simulink model "parts"  (R2021b)
settings: Solver=ode15s  StartTime=0.0  StopTime=t_f  MaxStep=max_step_size  RelTol=1e-3
values from neighbouring files (symbols this model uses):
  cont_param_10 = in    [double_pendulum.m]    (also in optimize_10_SMC_single_first_explicit.m = cont_param_10_surrogateopt)
  cont_param_11 = in    [double_pendulum.m]    (also in optimize_11_SMC_single_first_implicit.m = cont_param_11_surrogateopt)
  cont_param_12 = in    [double_pendulum.m]    (also in optimize_12_SMC_single_last_explicit.m = cont_param_12_surrogateopt)
  cont_param_13 = in    [double_pendulum.m]    (also in optimize_13_SMC_single_last_implicit.m = cont_param_13_surrogateopt)
  cont_param_14 = in    [double_pendulum.m]    (also in optimize_14_SMC_double_explicit.m = cont_param_14_surrogateopt)
  cont_param_15 = in    [double_pendulum.m]    (also in optimize_15_SMC_double_implicit.m = cont_param_15_surrogateopt)
  cont_param_16 = in    [double_pendulum.m]
  cont_param_17 = in    [double_pendulum.m]
  cont_param_18 = in    [double_pendulum.m]
  cont_param_19 = in    [double_pendulum.m]
  cont_param_4 = in    [double_pendulum.m]
  cont_param_5 = in    [double_pendulum.m]
  cont_param_6 = in    [double_pendulum.m]
  cont_param_7 = in    [double_pendulum.m]
  cont_param_8 = in    [double_pendulum.m]
  cont_param_9 = in    [double_pendulum.m]
  h = 1e-5    (= 1e-05)    [Conference_paper.m]    (also in Latest.m)
  m = 10    [Conference_paper.m]    (also in Latest.m = 100; control_8_collocated_PD_tracking.m = load_mass+hook_mass+cable_mass_total)
  method_select = Method    [main_run.m]    (also in modify_tracking.m = 3)
  N = floor(t_f / h)    [control_2_zero_vibration.m]    (also in control_3_ZVD.m; modify_tracking.m = 3)
  s = c1*(x-xd)+c2*(v-vd)+c3*theta_dot_1+c4*theta_1    [control_10_SMC_single_first_explicit.m]    (also in control_11_SMC_single_first_implicit.m = c1*(x-xd)+c2*(v-vd)+c3*theta_dot+c4*theta; control_12_SMC_single_last_explicit.m = c1*(x-xd)+c2*(v-vd)+c3*theta_dot_2+c4*theta_2; control_13_SMC_single_last_implicit.m = c1*(x-xd)+c2*(v-vd)+c3*theta_dot+c4*theta; control_14_SMC_double_explicit.m = (v-vd)+lambda*(x-xd)+alpha*theta_1+beta*theta_2)
  X = ex+lambda*sin(theta)    [control_16_PD_energy_first.m]    (also in control_17_PD_energy_last.m)
  Z = cont_param_8(4)    [control_8_collocated_PD_tracking.m]
undefined symbols (not defined in the file or in its folder): a_d_full, all_initial_sway, c_actuator, cable_eact_piece, cable_length, cable_mass_total, cart_disturbance_amp, cart_mass, delay_time, first_link_sway, hook_mass, last_piece_length, load_disturbance_amp, number_of_pendulums, payload_mass, sat_const, t_f, total_mass, traj_number, Y
libraries: sm_lib x72, nesl_utility x47, commchan3 x4
(part 1 of 2)
settings Model: Creator=rmoja  LastModifiedBy=SESA642626

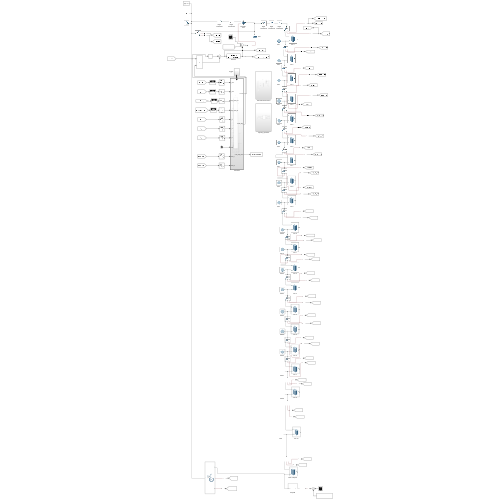
[thumbnail: Simulink's stored preview of the top-level diagram]
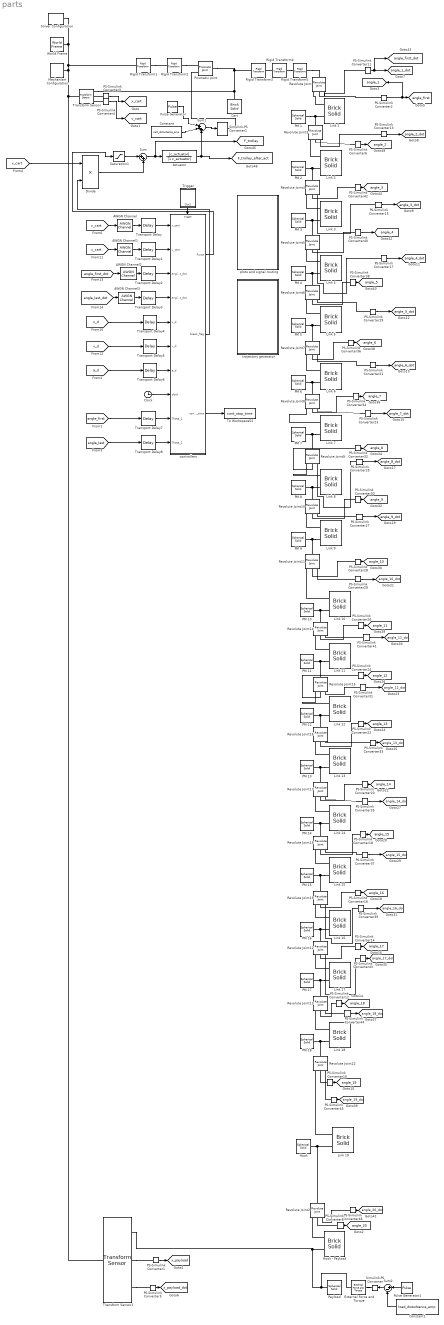
== system parts ==
  AWGN Channel{,1..3} (4 alike) : commchan3/AWGN Channel  InputProcessing=Columns as channels (frame based)  seed=67  noiseMode="Signal to noise ratio  (SNR)"  EbNodB=10  EsNodB=10  SNRdB=SNR_value  bitsPerSym=1  Ps=1  Tsym=1  variance=1
  Actuator : TransferFcn  Numerator=[c_actuator]  Denominator=[1 c_actuator]
  Cart : sm_lib/Body Elements/Brick Solid  GraphicAmbientColor=[0.15 0.15 0.15 1.0]  BasedOnType=Mass  BrickDimensions=[1/2 1/2 1/2]  BrickDimensionUnits=m  CenterOfMass=[0 0 0]  CenterOfMassUnits=m  GraphicDiffuseColor=[0 0 1]  Density=1000  DensityUnits=kg/(m^3)  DoExposeReferenceFrame=on  GraphicEmissiveColor=[0.0 0.0 0.0 1.0]  ExportEntireGeometry=off  SerializedFrames=<Frames/>  MarkerShape=Sphere  MarkerSize=10  GraphicType=FromGeometry  InertiaType=PointMass  Mass=cart_mass  MassUnits=kg  MomentsOfInertia=[1 1 1]  MomentsOfInertiaUnits=kg*m^2  GraphicOpacity=1.0  ProductsOfInertia=[0 0 0]  ProductsOfInertiaUnits=kg*m^2  GraphicShininess=75  GraphicSpecularColor=[0.5 0.5 0.5 1.0]  GraphicVisPropType=SimpleVisualProperties
  Clock : Clock
  Constant : Constant  Value=cart_disturbance_amp
  Constant1 : Constant  Value=load_disturbance_amp
  Divide : Product  Inputs=**
  External Force and Torque : sm_lib/Forces and Torques/External Force and Torque  ForceResolutionFrame=World  EnableForceX=on  EnableForceY=off  EnableForceZ=off  EnableForce=off  TorqueResolutionFrame=AttachedFrame  EnableTorqueX=off  EnableTorqueY=off  EnableTorqueZ=off  EnableTorque=off
  Hook : sm_lib/Body Elements/Spherical Solid  GraphicAmbientColor=[0.15 0.15 0.15 1.0]  BasedOnType=Density  CenterOfMass=[0 0 0]  CenterOfMassUnits=m  GraphicDiffuseColor=[1.0 0.2 0.0]  Density=1000  DensityUnits=kg/(m^3)  DoExposeReferenceFrame=on  GraphicEmissiveColor=[0.0 0.0 0.0 1.0]  ExportEntireGeometry=off  SerializedExposedGeometries=<ExposedGeometries/>  SerializedFrames=<Frames/>  MarkerShape=Sphere  MarkerSize=10  GraphicType=FromGeometry  InertiaType=PointMass  Mass=hook_mass-0.1  MassUnits=kg  MomentsOfInertia=[1 1 1]*1e-3  MomentsOfInertiaUnits=kg*m^2  GraphicOpacity=1.0  ProductsOfInertia=[0 0 0]  ProductsOfInertiaUnits=kg*m^2  GraphicShininess=75  GraphicSpecularColor=[0.5 0.5 0.5 1.0]  SphereRadius=0.2  SphereRadiusUnits=m  GraphicVisPropType=SimpleVisualProperties
  Hook - Payload : sm_lib/Body Elements/Brick Solid  GraphicAmbientColor=[0.15 0.15 0.15 1.0]  BasedOnType=Density  BrickDimensions=[last_piece_length 0.06 0.06]  BrickDimensionUnits=m  CenterOfMass=[0 0 0]  CenterOfMassUnits=m  GraphicDiffuseColor=[0.0 1 0.0]  Density=78000  DensityUnits=kg/m^3  DoExposeReferenceFrame=on  GraphicEmissiveColor=[0.0 0.0 0.0 1.0]  ExportEntireGeometry=off  SerializedFrames=<Frames><Frame><Id>Frame1</Id><Value><Name>F1</Name><Origin><Source>GeometricFeature</Source><FeatureName>-x surface</FeatureName></Origin><PrimaryAxis><DefinedDirection>+Z</DefinedDirection><Source>ReferenceFrame</Source><SourceDirection>+Z</SourceDirection><FeatureName></FeatureName></PrimaryAxis><SecondaryAxis><DefinedDirection>+X</DefinedDirection><Source>ReferenceFrame</Source><SourceDirection>+X</SourceDirection><FeatureName></FeatureName></SecondaryAxis></Value></Frame><Frame><Id>Frame2</Id><Value><Name>F2</Name><Origin><Source>GeometricFeature</Source><FeatureName>+x surface</FeatureName></Origin><PrimaryAxis><DefinedDirection>+Z</DefinedDirection><Source>ReferenceFrame</Source><SourceDirection>+Z</SourceDirection><FeatureName></FeatureName></PrimaryAxis><SecondaryAxis><DefinedDirection>+X</DefinedDirection><Source>ReferenceFrame</Source><SourceDirection>+X</SourceDirection><FeatureName></FeatureName></SecondaryAxis></Value></Frame></Frames>  MarkerShape=Sphere  MarkerSize=10  GraphicType=FromGeometry  InertiaType=PointMass  Mass=0  MassUnits=kg  MomentsOfInertia=[1 1 1]  MomentsOfInertiaUnits=kg*m^2  GraphicOpacity=1.0  ProductsOfInertia=[0 0 0]  ProductsOfInertiaUnits=kg*m^2  GraphicShininess=75  GraphicSpecularColor=[0.5 0.5 0.5 1.0]  GraphicVisPropType=SimpleVisualProperties
  Link {1..18} (18 alike) : sm_lib/Body Elements/Brick Solid  GraphicAmbientColor=[0.15 0.15 0.15 1.0]  BasedOnType=Mass  BrickDimensions=[cable_length/number_of_pendulums 0.02 0.02]  BrickDimensionUnits=m  CenterOfMass=[0 0 0]  CenterOfMassUnits=m  GraphicDiffuseColor=[0 0 0]  Density=7800  DensityUnits=kg/m^3  DoExposeReferenceFrame=on  GraphicEmissiveColor=[0.0 0.0 0.0 1.0]  ExportEntireGeometry=off  SerializedFrames=<Frames><Frame><Id>Frame1</Id><Value><Name>F1</Name><Origin><Source>GeometricFeature</Source><FeatureName>-x surface</FeatureName></Origin><PrimaryAxis><DefinedDirection>+Z</DefinedDirection><Source>ReferenceFrame</Source><SourceDirection>+Z</SourceDirection><FeatureName></FeatureName></PrimaryAxis><SecondaryAxis><DefinedDirection>+X</DefinedDirection><Source>ReferenceFrame</Source><SourceDirection>+X</SourceDirection><FeatureName></FeatureName></SecondaryAxis></Value></Frame><Frame><Id>Frame2</Id><Value><Name>F2</Name><Origin><Source>GeometricFeature</Source><FeatureName>+x surface</FeatureName></Origin><PrimaryAxis><DefinedDirection>+Z</DefinedDirection><Source>ReferenceFrame</Source><SourceDirection>+Z</SourceDirection><FeatureName></FeatureName></PrimaryAxis><SecondaryAxis><DefinedDirection>+X</DefinedDirection><Source>ReferenceFrame</Source><SourceDirection>+X</SourceDirection><FeatureName></FeatureName></SecondaryAxis></Value></Frame></Frames>  MarkerShape=Sphere  MarkerSize=10  GraphicType=FromGeometry  InertiaType=PointMass  Mass=0  MassUnits=kg  MomentsOfInertia=[1 1 1]  MomentsOfInertiaUnits=kg*m^2  GraphicOpacity=1.0  ProductsOfInertia=[0 0 0]  ProductsOfInertiaUnits=kg*m^2  GraphicShininess=75  GraphicSpecularColor=[0.5 0.5 0.5 1.0]  GraphicVisPropType=SimpleVisualProperties
  Link 19 : sm_lib/Body Elements/Brick Solid  GraphicAmbientColor=[0.15 0.15 0.15 1.0]  BasedOnType=Mass  BrickDimensions=[cable_length/number_of_pendulums 0.02 0.02]  BrickDimensionUnits=m  CenterOfMass=[0 0 0]  CenterOfMassUnits=m  GraphicDiffuseColor=[0 0 0]  Density=7800  DensityUnits=kg/m^3  DoExposeReferenceFrame=on  GraphicEmissiveColor=[0.0 0.0 0.0 1.0]  ExportEntireGeometry=off  SerializedFrames=<Frames><Frame><Id>Frame1</Id><Value><Name>F1</Name><Origin><Source>GeometricFeature</Source><FeatureName>-x surface</FeatureName></Origin><PrimaryAxis><DefinedDirection>+Z</DefinedDirection><Source>ReferenceFrame</Source><SourceDirection>+Z</SourceDirection><FeatureName></FeatureName></PrimaryAxis><SecondaryAxis><DefinedDirection>+X</DefinedDirection><Source>ReferenceFrame</Source><SourceDirection>+X</SourceDirection><FeatureName></FeatureName></SecondaryAxis></Value></Frame><Frame><Id>Frame2</Id><Value><Name>F2</Name><Origin><Source>GeometricFeature</Source><FeatureName>+x surface</FeatureName></Origin><PrimaryAxis><DefinedDirection>+Z</DefinedDirection><Source>ReferenceFrame</Source><SourceDirection>+Z</SourceDirection><FeatureName></FeatureName></PrimaryAxis><SecondaryAxis><DefinedDirection>+X</DefinedDirection><Source>ReferenceFrame</Source><SourceDirection>+X</SourceDirection><FeatureName></FeatureName></SecondaryAxis></Value></Frame></Frames>  MarkerShape=Sphere  MarkerSize=10  GraphicType=FromGeometry  InertiaType=PointMass  Mass=0.1  MassUnits=kg  MomentsOfInertia=[1 1 1]  MomentsOfInertiaUnits=kg*m^2  GraphicOpacity=1.0  ProductsOfInertia=[0 0 0]  ProductsOfInertiaUnits=kg*m^2  GraphicShininess=75  GraphicSpecularColor=[0.5 0.5 0.5 1.0]  GraphicVisPropType=SimpleVisualProperties
  Mechanism Configuration : sm_lib/Utilities/Mechanism Configuration  UniformGravity=Constant  GravityVector=[0 0 -9.80665]  GravityUnits=m/s^2  LinearizationDelta=0.001  JointModeTransitionNonlinearIterations=2
  PM {1..18} (18 alike) : sm_lib/Body Elements/Spherical Solid  GraphicAmbientColor=[0.15 0.15 0.15 1.0]  BasedOnType=Density  CenterOfMass=[0 0 0]  CenterOfMassUnits=m  GraphicDiffuseColor=[1.0 0.2 0.0]  Density=1000  DensityUnits=kg/(m^3)  DoExposeReferenceFrame=on  GraphicEmissiveColor=[0.0 0.0 0.0 1.0]  ExportEntireGeometry=off  SerializedExposedGeometries=<ExposedGeometries/>  SerializedFrames=<Frames/>  MarkerShape=Sphere  MarkerSize=10  GraphicType=FromGeometry  InertiaType=PointMass  Mass=cable_eact_piece  MassUnits=kg  MomentsOfInertia=[1 1 1]*1e-3  MomentsOfInertiaUnits=kg*m^2  GraphicOpacity=1.0  ProductsOfInertia=[0 0 0]  ProductsOfInertiaUnits=kg*m^2  GraphicShininess=75  GraphicSpecularColor=[0.5 0.5 0.5 1.0]  SphereRadius=0.05  SphereRadiusUnits=m  GraphicVisPropType=SimpleVisualProperties
  PS-Simulink Converter{1..6,8,10..46} (44 alike) : nesl_utility/PS-Simulink Converter  PhysicalDomain=network_engine_domain  SubClassName=ps_output  LeftPortType=input  RightPortType=output  PseudoPeriodic=off  Frequencies=[]  Unit=inherit  AffineConversion=off
      settings: SourceProductBaseCode=PW,SS
  Payload : sm_lib/Body Elements/Spherical Solid  GraphicAmbientColor=[0.15 0.15 0.15 1.0]  BasedOnType=Density  CenterOfMass=[0 0 0]  CenterOfMassUnits=m  GraphicDiffuseColor=[1.0 0.2 0.0]  Density=1000  DensityUnits=kg/(m^3)  DoExposeReferenceFrame=on  GraphicEmissiveColor=[0.0 0.0 0.0 1.0]  ExportEntireGeometry=off  SerializedExposedGeometries=<ExposedGeometries/>  SerializedFrames=<Frames><Frame><Id>Frame1</Id><Value><Name>F1</Name><Origin><Source>ReferenceFrame</Source><FeatureName></FeatureName></Origin><PrimaryAxis><DefinedDirection>+Z</DefinedDirection><Source>ReferenceFrame</Source><SourceDirection>+Z</SourceDirection><FeatureName></FeatureName></PrimaryAxis><SecondaryAxis><DefinedDirection>+X</DefinedDirection><Source>ReferenceFrame</Source><SourceDirection>+X</SourceDirection><FeatureName></FeatureName></SecondaryAxis></Value></Frame></Frames>  MarkerShape=Sphere  MarkerSize=10  GraphicType=FromGeometry  InertiaType=PointMass  Mass=payload_mass  MassUnits=kg  MomentsOfInertia=[1 1 1]*1e-3  MomentsOfInertiaUnits=kg*m^2  GraphicOpacity=1.0  ProductsOfInertia=[0 0 0]  ProductsOfInertiaUnits=kg*m^2  GraphicShininess=75  GraphicSpecularColor=[0.5 0.5 0.5 1.0]  SphereRadius=0.4  SphereRadiusUnits=m  GraphicVisPropType=SimpleVisualProperties
  Prismatic Joint : sm_lib/Joints/Prismatic Joint  JointMode=Normal  SenseConstraintForce=off  SenseConstraintForceX=off  SenseConstraintForceY=off  SenseConstraintForceZ=off  SenseConstraintTorque=off  SenseConstraintTorqueX=off  SenseConstraintTorqueY=off  SenseConstraintTorqueZ=off  SenseTotalForce=off  SenseTotalForceX=off  SenseTotalForceY=off  SenseTotalForceZ=off  SenseTotalTorque=off  SenseTotalTorqueX=off  SenseTotalTorqueY=off  SenseTotalTorqueZ=off  CompositeWrenchDir=FollowerOnBase  CompositeWrenchFrame=BaseFrame  EquilibriumPosition=0  EquilibriumPositionUnits=m  SpringStiffness=0  SpringStiffnessUnits=N/m  DampingCoefficient=0  DampingCoefficientUnits=N/(m/s)  TorqueActuationMode=InputTorque  MotionActuationMode=ComputedMotion  SensePosition=off  SenseVelocity=off  SenseAcceleration=off  SenseTorqueForce=off  SenseLowerLimitTorqueForce=off  SenseUpperLimitTorqueForce=off  LowerLimitSpecify=off  LowerLimitBound=-1  LowerLimitBoundUnits=m  LowerLimitStiffness=1e6  LowerLimitStiffnessUnits=N/m  LowerLimitDamping=1e3  LowerLimitDampingUnits=N/(m/s)  LowerLimitTransitionRegionWidth=1e-4  LowerLimitTransitionRegionWidthUnits=m  UpperLimitSpecify=off  UpperLimitBound=1  UpperLimitBoundUnits=m  UpperLimitStiffness=1e6  UpperLimitStiffnessUnits=N/m  UpperLimitDamping=1e3  UpperLimitDampingUnits=N/(m/s)  UpperLimitTransitionRegionWidth=1e-4  UpperLimitTransitionRegionWidthUnits=m  PositionTargetSpecify=off  PositionTargetPriority=High  PositionTargetValue=0  PositionTargetValueUnits=m  VelocityTargetSpecify=off  VelocityTargetPriority=High  VelocityTargetValue=0  VelocityTargetValueUnits=m/s
  Pulse Generator : DiscretePulseGenerator  PulseType=Time based  Amplitude=2*cart_disturbance_amp  Period=20  PulseWidth=50
  Pulse Generator1 : DiscretePulseGenerator  PulseType=Time based  Amplitude=2*load_disturbance_amp  Period=20  PulseWidth=50
  Revolute Joint : sm_lib/Joints/Revolute Joint  JointMode=Normal  SenseConstraintForce=off  SenseConstraintForceX=off  SenseConstraintForceY=off  SenseConstraintForceZ=off  SenseConstraintTorque=off  SenseConstraintTorqueX=off  SenseConstraintTorqueY=off  SenseConstraintTorqueZ=off  SenseTotalForce=off  SenseTotalForceX=off  SenseTotalForceY=off  SenseTotalForceZ=off  SenseTotalTorque=off  SenseTotalTorqueX=off  SenseTotalTorqueY=off  SenseTotalTorqueZ=off  CompositeWrenchDir=FollowerOnBase  CompositeWrenchFrame=BaseFrame  EquilibriumPosition=0  EquilibriumPositionUnits=deg  SpringStiffness=joint_stiffness  SpringStiffnessUnits=N*m/deg  DampingCoefficient=damping_coefficient  DampingCoefficientUnits=N*m/(deg/s)  TorqueActuationMode=NoTorque  MotionActuationMode=ComputedMotion  SensePosition=on  SenseVelocity=on  SenseAcceleration=off  SenseTorqueForce=off  SenseLowerLimitTorqueForce=off  SenseUpperLimitTorqueForce=off  LowerLimitSpecify=off  LowerLimitBound=-90  LowerLimitBoundUnits=deg  LowerLimitStiffness=1e4  LowerLimitStiffnessUnits=N*m/deg  LowerLimitDamping=10  LowerLimitDampingUnits=N*m/(deg/s)  LowerLimitTransitionRegionWidth=0.1  LowerLimitTransitionRegionWidthUnits=deg  UpperLimitSpecify=off  UpperLimitBound=90  UpperLimitBoundUnits=deg  UpperLimitStiffness=1e4  UpperLimitStiffnessUnits=N*m/deg  UpperLimitDamping=10  UpperLimitDampingUnits=N*m/(deg/s)  UpperLimitTransitionRegionWidth=0.1  UpperLimitTransitionRegionWidthUnits=deg  PositionTargetSpecify=on  PositionTargetPriority=High  PositionTargetValue=first_link_sway+all_initial_sway  PositionTargetValueUnits=deg  VelocityTargetSpecify=off  VelocityTargetPriority=High  VelocityTargetValue=0  VelocityTargetValueUnits=deg/s
  Revolute Joint{4,6,8,10,12,14,16,18,22} (9 alike) : sm_lib/Joints/Revolute Joint  JointMode=Normal  SenseConstraintForce=off  SenseConstraintForceX=off  SenseConstraintForceY=off  SenseConstraintForceZ=off  SenseConstraintTorque=off  SenseConstraintTorqueX=off  SenseConstraintTorqueY=off  SenseConstraintTorqueZ=off  SenseTotalForce=off  SenseTotalForceX=off  SenseTotalForceY=off  SenseTotalForceZ=off  SenseTotalTorque=off  SenseTotalTorqueX=off  SenseTotalTorqueY=off  SenseTotalTorqueZ=off  CompositeWrenchDir=FollowerOnBase  CompositeWrenchFrame=BaseFrame  EquilibriumPosition=0  EquilibriumPositionUnits=deg  SpringStiffness=joint_stiffness  SpringStiffnessUnits=N*m/deg  DampingCoefficient=damping_coefficient  DampingCoefficientUnits=N*m/(deg/s)  TorqueActuationMode=NoTorque  MotionActuationMode=ComputedMotion  SensePosition=on  SenseVelocity=on  SenseAcceleration=off  SenseTorqueForce=off  SenseLowerLimitTorqueForce=off  SenseUpperLimitTorqueForce=off  LowerLimitSpecify=off  LowerLimitBound=-90  LowerLimitBoundUnits=deg  LowerLimitStiffness=1e4  LowerLimitStiffnessUnits=N*m/deg  LowerLimitDamping=10  LowerLimitDampingUnits=N*m/(deg/s)  LowerLimitTransitionRegionWidth=0.1  LowerLimitTransitionRegionWidthUnits=deg  UpperLimitSpecify=off  UpperLimitBound=90  UpperLimitBoundUnits=deg  UpperLimitStiffness=1e4  UpperLimitStiffnessUnits=N*m/deg  UpperLimitDamping=10  UpperLimitDampingUnits=N*m/(deg/s)  UpperLimitTransitionRegionWidth=0.1  UpperLimitTransitionRegionWidthUnits=deg  PositionTargetSpecify=on  PositionTargetPriority=High  PositionTargetValue=all_initial_sway  PositionTargetValueUnits=deg  VelocityTargetSpecify=off  VelocityTargetPriority=High  VelocityTargetValue=0  VelocityTargetValueUnits=deg/s
  Revolute Joint{3,5,7,9,11,13,15,17,19} (9 alike) : sm_lib/Joints/Revolute Joint  JointMode=Normal  SenseConstraintForce=off  SenseConstraintForceX=off  SenseConstraintForceY=off  SenseConstraintForceZ=off  SenseConstraintTorque=off  SenseConstraintTorqueX=off  SenseConstraintTorqueY=off  SenseConstraintTorqueZ=off  SenseTotalForce=off  SenseTotalForceX=off  SenseTotalForceY=off  SenseTotalForceZ=off  SenseTotalTorque=off  SenseTotalTorqueX=off  SenseTotalTorqueY=off  SenseTotalTorqueZ=off  CompositeWrenchDir=FollowerOnBase  CompositeWrenchFrame=BaseFrame  EquilibriumPosition=0  EquilibriumPositionUnits=deg  SpringStiffness=joint_stiffness  SpringStiffnessUnits=N*m/deg  DampingCoefficient=damping_coefficient  DampingCoefficientUnits=N*m/(deg/s)  TorqueActuationMode=NoTorque  MotionActuationMode=ComputedMotion  SensePosition=on  SenseVelocity=on  SenseAcceleration=off  SenseTorqueForce=off  SenseLowerLimitTorqueForce=off  SenseUpperLimitTorqueForce=off  LowerLimitSpecify=off  LowerLimitBound=-90  LowerLimitBoundUnits=deg  LowerLimitStiffness=1e4  LowerLimitStiffnessUnits=N*m/deg  LowerLimitDamping=10  LowerLimitDampingUnits=N*m/(deg/s)  LowerLimitTransitionRegionWidth=0.1  LowerLimitTransitionRegionWidthUnits=deg  UpperLimitSpecify=off  UpperLimitBound=90  UpperLimitBoundUnits=deg  UpperLimitStiffness=1e4  UpperLimitStiffnessUnits=N*m/deg  UpperLimitDamping=10  UpperLimitDampingUnits=N*m/(deg/s)  UpperLimitTransitionRegionWidth=0.1  UpperLimitTransitionRegionWidthUnits=deg  PositionTargetSpecify=on  PositionTargetPriority=High  PositionTargetValue=-all_initial_sway  PositionTargetValueUnits=deg  VelocityTargetSpecify=off  VelocityTargetPriority=High  VelocityTargetValue=0  VelocityTargetValueUnits=deg/s
  Revolute Joint2 : sm_lib/Joints/Revolute Joint  JointMode=Normal  SenseConstraintForce=off  SenseConstraintForceX=off  SenseConstraintForceY=off  SenseConstraintForceZ=off  SenseConstraintTorque=off  SenseConstraintTorqueX=off  SenseConstraintTorqueY=off  SenseConstraintTorqueZ=off  SenseTotalForce=off  SenseTotalForceX=off  SenseTotalForceY=off  SenseTotalForceZ=off  SenseTotalTorque=off  SenseTotalTorqueX=off  SenseTotalTorqueY=off  SenseTotalTorqueZ=off  CompositeWrenchDir=FollowerOnBase  CompositeWrenchFrame=BaseFrame  EquilibriumPosition=0  EquilibriumPositionUnits=deg  SpringStiffness=0  SpringStiffnessUnits=N*m/deg  DampingCoefficient=damping_coefficient  DampingCoefficientUnits=N*m/(deg/s)  TorqueActuationMode=NoTorque  MotionActuationMode=ComputedMotion  SensePosition=on  SenseVelocity=on  SenseAcceleration=off  SenseTorqueForce=off  SenseLowerLimitTorqueForce=off  SenseUpperLimitTorqueForce=off  LowerLimitSpecify=off  LowerLimitBound=-90  LowerLimitBoundUnits=deg  LowerLimitStiffness=1e4  LowerLimitStiffnessUnits=N*m/deg  LowerLimitDamping=10  LowerLimitDampingUnits=N*m/(deg/s)  LowerLimitTransitionRegionWidth=0.1  LowerLimitTransitionRegionWidthUnits=deg  UpperLimitSpecify=off  UpperLimitBound=90  UpperLimitBoundUnits=deg  UpperLimitStiffness=1e4  UpperLimitStiffnessUnits=N*m/deg  UpperLimitDamping=10  UpperLimitDampingUnits=N*m/(deg/s)  UpperLimitTransitionRegionWidth=0.1  UpperLimitTransitionRegionWidthUnits=deg  PositionTargetSpecify=on  PositionTargetPriority=High  PositionTargetValue=-all_initial_sway  PositionTargetValueUnits=deg  VelocityTargetSpecify=off  VelocityTargetPriority=High  VelocityTargetValue=0  VelocityTargetValueUnits=deg/s
  Rigid Transform1 : sm_lib/Frames and Transforms/Rigid Transform  TranslationMethod=None  TranslationStandardOffset=0  TranslationLengthUnit=m  TranslationStandardAxis=+Z  TranslationCartesianOffset=[0 0 0]  TranslationROffset=0  TranslationROffsetUnits=m  TranslationZOffset=0  TranslationZOffsetUnits=m  TranslationThetaOffset=0  TranslationThetaOffsetUnits=deg  RotationMethod=StandardAxis  RotationAngleUnits=deg  RotationStandardAxis=+Y  RotationAngle=90  RotationArbitraryAxis=[0 0 1]  FollAlignAxisA=+X  BaseAlignAxisA=+Y  FollAlignAxisB=+Y  BaseAlignAxisB=+Z  RotationSequenceAxes=FollowerAxes  RotationSequence=XYX  RotationSequenceAngles=[0 0 0]  RotationSequenceAnglesUnits=deg  RotationMatrix=[1 0 0; 0 1 0; 0 0 1]
  Rigid Transform2 : sm_lib/Frames and Transforms/Rigid Transform  TranslationMethod=None  TranslationStandardOffset=0  TranslationLengthUnit=m  TranslationStandardAxis=+Z  TranslationCartesianOffset=[0 0 0]  TranslationROffset=0  TranslationROffsetUnits=m  TranslationZOffset=0  TranslationZOffsetUnits=m  TranslationThetaOffset=0  TranslationThetaOffsetUnits=deg  RotationMethod=StandardAxis  RotationAngleUnits=deg  RotationStandardAxis=+Z  RotationAngle=180  RotationArbitraryAxis=[0 0 1]  FollAlignAxisA=+X  BaseAlignAxisA=+Y  FollAlignAxisB=+Y  BaseAlignAxisB=+Z  RotationSequenceAxes=FollowerAxes  RotationSequence=XYX  RotationSequenceAngles=[0 0 0]  RotationSequenceAnglesUnits=deg  RotationMatrix=[1 0 0; 0 1 0; 0 0 1]
  Rigid Transform3 : sm_lib/Frames and Transforms/Rigid Transform  TranslationMethod=None  TranslationStandardOffset=0  TranslationLengthUnit=m  TranslationStandardAxis=+Z  TranslationCartesianOffset=[0 0 0]  TranslationROffset=0  TranslationROffsetUnits=m  TranslationZOffset=0  TranslationZOffsetUnits=m  TranslationThetaOffset=0  TranslationThetaOffsetUnits=deg  RotationMethod=StandardAxis  RotationAngleUnits=deg  RotationStandardAxis=-X  RotationAngle=90  RotationArbitraryAxis=[0 0 1]  FollAlignAxisA=+X  BaseAlignAxisA=+Y  FollAlignAxisB=+Y  BaseAlignAxisB=+Z  RotationSequenceAxes=FollowerAxes  RotationSequence=XYX  RotationSequenceAngles=[0 0 0]  RotationSequenceAnglesUnits=deg  RotationMatrix=[1 0 0; 0 1 0; 0 0 1]
  Rigid Transform4 : sm_lib/Frames and Transforms/Rigid Transform  TranslationMethod=None  TranslationStandardOffset=0  TranslationLengthUnit=m  TranslationStandardAxis=+Z  TranslationCartesianOffset=[0 0 0]  TranslationROffset=0  TranslationROffsetUnits=m  TranslationZOffset=0  TranslationZOffsetUnits=m  TranslationThetaOffset=0  TranslationThetaOffsetUnits=deg  RotationMethod=StandardAxis  RotationAngleUnits=deg  RotationStandardAxis=+Y  RotationAngle=180  RotationArbitraryAxis=[0 0 1]  FollAlignAxisA=+X  BaseAlignAxisA=+Y  FollAlignAxisB=+Y  BaseAlignAxisB=+Z  RotationSequenceAxes=FollowerAxes  RotationSequence=XYX  RotationSequenceAngles=[0 0 0]  RotationSequenceAnglesUnits=deg  RotationMatrix=[1 0 0; 0 1 0; 0 0 1]
  Rigid Transform5 : sm_lib/Frames and Transforms/Rigid Transform  TranslationMethod=None  TranslationStandardOffset=0  TranslationLengthUnit=m  TranslationStandardAxis=+Z  TranslationCartesianOffset=[0 0 0]  TranslationROffset=0  TranslationROffsetUnits=m  TranslationZOffset=0  TranslationZOffsetUnits=m  TranslationThetaOffset=0  TranslationThetaOffsetUnits=deg  RotationMethod=StandardAxis  RotationAngleUnits=deg  RotationStandardAxis=+X  RotationAngle=180  RotationArbitraryAxis=[0 0 1]  FollAlignAxisA=+X  BaseAlignAxisA=+Y  FollAlignAxisB=+Y  BaseAlignAxisB=+Z  RotationSequenceAxes=FollowerAxes  RotationSequence=XYX  RotationSequenceAngles=[0 0 0]  RotationSequenceAnglesUnits=deg  RotationMatrix=[1 0 0; 0 1 0; 0 0 1]
  Saturation1 : Saturate  UpperLimit=+sat_const  LowerLimit=-sat_const
  Simulink-PS Converter : nesl_utility/Simulink-PS Converter  PhysicalDomain=network_engine_domain  SubClassName=ps_input  LeftPortType=input  RightPortType=output  PseudoPeriodic=off  Frequencies=[]  NoiseDistribution=none  NoiseParameters=[]  Unit=1  AffineConversion=off  FilteringAndDerivatives=provide  SimscapeFilterOrder=1  InputFilterTimeConstant=0.001  UdotUserProvided=0
      settings: SourceProductBaseCode=PW,SS
  Simulink-PS Converter1 : nesl_utility/Simulink-PS Converter  PhysicalDomain=network_engine_domain  SubClassName=ps_input  LeftPortType=input  RightPortType=output  PseudoPeriodic=off  Frequencies=[]  NoiseDistribution=none  NoiseParameters=[]  Unit=1  AffineConversion=off  FilteringAndDerivatives=zero  SimscapeFilterOrder=1  InputFilterTimeConstant=0.001  UdotUserProvided=1
      settings: SourceProductBaseCode=PW,SS
  Solver Configuration : nesl_utility/Solver Configuration  PhysicalDomain=network_engine_domain  SubClassName=solver  LeftPortType=input  RightPortType=generic  Tones=[]  Harmonics=[]  SimulateNoise=off  Profile=off  UseLocalSampling=off  EnableSwitchedLinearOptims=on  FrequencyDomain=off  UseCCode=off  RelTol=0.001  AbsTol=1e-06  MinStep=1e-09  ToWorkspace=off  RevertToSquareIcSolve=off  NumHomotopyIterations=100  PhasorMode=off  PhasorModeNumHarmonics=1  DoDC=off  ResidualTolerance=1e-09  UseLocalSolver=off  LocalSolverChoice=NE_BACKWARD_EULER_ADVANCER  LocalSolverSampleTime=0.001  DoFixedCost=off  MaxNonlinIter=3  MaxModeIter=2  ComputeImpulses=off  ImpulseIterations=2  LinearAlgebra=auto  EquationFormulation=NE_TIME_EF  DelaysMemoryBudget=1024  AutomaticFiltering=on  FilteringTimeConstant=0.001  PartitionStorageMethod=AS_NEEDED  PartitionMemoryBudget=1024  PartitionMethod=ROBUST
      settings: SourceProductBaseCode=PW,SS
  Sum : Sum  Inputs=|++
  Sum1 : Sum  Inputs=|+-+
  Sum2 : Sum  Inputs=|+-
  To Workspace52 : ToWorkspace  VariableName=cont_stop_time  SampleTime=-1
  Transform Sensor : sm_lib/Frames and Transforms/Transform Sensor  MeasurementFrame=World  SenseAngle=off  SenseAxis=off  SenseAngle1=off  SenseAngle2=off  SenseAngle3=off  SenseQ=off  SenseR=off  SenseOmegaX=off  SenseOmegaY=off  SenseOmegaZ=off  SenseOmega1=off  SenseOmega2=off  SenseOmega3=off  SenseQDot=off  SenseRDot=off  SenseAlphaX=off  SenseAlphaY=off  SenseAlphaZ=off  SenseAlpha1=off  SenseAlpha2=off  SenseAlpha3=off  SenseQDDot=off  SenseRDDot=off  SenseX=on  SenseY=off  SenseZ=off  SenseRad=off  SenseAzim=off  SenseDist=off  SenseInc=off  SenseXDot=on  SenseYDot=off  SenseZDot=off  SenseRadDot=off  SenseAzimDot=off  SenseDistDot=off  SenseIncDot=off  SenseXDDot=off  SenseYDDot=off  SenseZDDot=off  SenseRadDDot=off  SenseAzimDDot=off  SenseDistDDot=off  SenseIncDDot=off
  Transform Sensor1 : sm_lib/Frames and Transforms/Transform Sensor  MeasurementFrame=World  SenseAngle=off  SenseAxis=off  SenseAngle1=off  SenseAngle2=off  SenseAngle3=off  SenseQ=off  SenseR=off  SenseOmegaX=off  SenseOmegaY=off  SenseOmegaZ=off  SenseOmega1=off  SenseOmega2=off  SenseOmega3=off  SenseQDot=off  SenseRDot=off  SenseAlphaX=off  SenseAlphaY=off  SenseAlphaZ=off  SenseAlpha1=off  SenseAlpha2=off  SenseAlpha3=off  SenseQDDot=off  SenseRDDot=off  SenseX=on  SenseY=off  SenseZ=off  SenseRad=off  SenseAzim=off  SenseDist=off  SenseInc=off  SenseXDot=on  SenseYDot=off  SenseZDot=off  SenseRadDot=off  SenseAzimDot=off  SenseDistDot=off  SenseIncDot=off  SenseXDDot=off  SenseYDDot=off  SenseZDDot=off  SenseRadDDot=off  SenseAzimDDot=off  SenseDistDDot=off  SenseIncDDot=off
  Transport Delay{,1..8} (9 alike) : TransportDelay  DelayTime=delay_time
  Trigger : Subsystem
  World Frame : sm_lib/Frames and Transforms/World Frame
  controllers : Subsystem  TreatAsAtomicUnit=on
  plots and signal routing : Subsystem
  trajectory generator : Subsystem
  tag scope: F_trolley=global, F_trolley_after_act=global, angle_10=global, angle_10_dot=global, angle_11=global, angle_11_dot=global, angle_12=global, angle_12_dot=global, angle_13=global, angle_13_dot=global, angle_14=global, angle_14_dot=global, angle_15=global, angle_15_dot=global, angle_16=global, angle_16_dot=global, angle_17=global, angle_17_dot=global, angle_18=global, angle_18_dot=global, angle_19=global, angle_19_dot=global, angle_1=global, angle_1_dot=global, angle_20=global, angle_20_dot=global, angle_2=global, angle_2_dot=global, angle_3=global, angle_3_dot=global, angle_4=global, angle_4_dot=global, angle_5=global, angle_5_dot=global, angle_6=global, angle_6_dot=global, angle_7=global, angle_7_dot=global, angle_8=global, angle_8_dot=global, angle_9=global, angle_9_dot=global, angle_first=global, angle_first_dot=global, v_cart=global, x_cart=global, x_payload=global, x_payload_dot=global
  wires:
  PS-Simulink Converter3/1 -> [x_cart]
  PS-Simulink Converter4/1 -> [v_cart]
  PS-Simulink Converter1/1 -> [x_payload]
  PS-Simulink Converter5/1 -> [x_payload_dot]
  PS-Simulink Converter6/1 -> [angle_2]
  PS-Simulink Converter8/1 -> [angle_20]
  PS-Simulink Converter10/1 -> [angle_19]
  PS-Simulink Converter12/1 -> [angle_18]
  PS-Simulink Converter14/1 -> [angle_17]
  PS-Simulink Converter16/1 -> [angle_16]
  PS-Simulink Converter18/1 -> [angle_15]
  PS-Simulink Converter20/1 -> [angle_14]
  PS-Simulink Converter22/1 -> [angle_13]
  PS-Simulink Converter24/1 -> [angle_12]
  PS-Simulink Converter26/1 -> [angle_11]
  PS-Simulink Converter28/1 -> [angle_10]
  PS-Simulink Converter30/1 -> [angle_9]
  PS-Simulink Converter32/1 -> [angle_8]
  PS-Simulink Converter34/1 -> [angle_7]
  PS-Simulink Converter36/1 -> [angle_6]
  PS-Simulink Converter38/1 -> [angle_5]
  PS-Simulink Converter40/1 -> [angle_4]
  PS-Simulink Converter42/1 -> [angle_3]
  PS-Simulink Converter2/1 -> [angle_1], [angle_first]
  PS-Simulink Converter11/1 -> [angle_first_dot], [angle_1_dot]
  PS-Simulink Converter13/1 -> [angle_2_dot]
  PS-Simulink Converter15/1 -> [angle_3_dot]
  PS-Simulink Converter17/1 -> [angle_4_dot]
  PS-Simulink Converter19/1 -> [angle_5_dot]
  PS-Simulink Converter21/1 -> [angle_6_dot]
  PS-Simulink Converter23/1 -> [angle_7_dot]
  PS-Simulink Converter25/1 -> [angle_8_dot]
  PS-Simulink Converter27/1 -> [angle_9_dot]
  PS-Simulink Converter29/1 -> [angle_10_dot]
  PS-Simulink Converter35/1 -> [angle_14_dot]
  PS-Simulink Converter37/1 -> [angle_15_dot]
  PS-Simulink Converter39/1 -> [angle_16_dot]
  PS-Simulink Converter41/1 -> [angle_11_dot]
  PS-Simulink Converter31/1 -> [angle_12_dot]
  PS-Simulink Converter33/1 -> [angle_13_dot]
  PS-Simulink Converter43/1 -> [angle_17_dot]
  PS-Simulink Converter44/1 -> [angle_18_dot]
  PS-Simulink Converter45/1 -> [angle_19_dot]
  PS-Simulink Converter46/1 -> [angle_20_dot]
  [v_cart] -> AWGN Channel1/1
  Trigger/1(Out1) -> controllers/Trigger
  Clock/1 -> controllers/8(clock)
  [angle_first] -> Transport Delay7/1
  [angle_last] -> Transport Delay8/1
  [x_cart] -> AWGN Channel/1
  Transport Delay/1 -> controllers/1(x_cart)
  Transport Delay1/1 -> controllers/2(v_cart)
  Transport Delay2/1 -> controllers/3(angle_first_dot)
  Transport Delay3/1 -> controllers/4(angle_last_dot)
  Transport Delay4/1 -> controllers/5(x_d)
  Transport Delay5/1 -> controllers/6(v_d)
  Transport Delay6/1 -> controllers/7(a_d)
  Transport Delay7/1 -> controllers/9(Theta_1)
  Transport Delay8/1 -> controllers/10(Theta_2)
  controllers/1(Force) -> Saturation1/1
  [v_cart] -> Divide/1
  controllers/2(break_flag) -> Divide/2
  controllers/3(cont_stop_time) -> To Workspace52/1
  AWGN Channel/1 -> Transport Delay/1
  AWGN Channel1/1 -> Transport Delay1/1
  [angle_first_dot] -> AWGN Channel2/1
  AWGN Channel2/1 -> Transport Delay2/1
  AWGN Channel3/1 -> Transport Delay3/1
  [angle_last_dot] -> AWGN Channel3/1
  [x_d] -> Transport Delay4/1
  [v_d] -> Transport Delay5/1
  [a_d] -> Transport Delay6/1
  Sum/1 -> Actuator/1, [F_trolley]
  Actuator/1 -> Sum1/3, [F_trolley_after_act]
  Saturation1/1 -> Sum/1
  Divide/1 -> Sum/2
  Sum1/1 -> Simulink-PS Converter1/1
  Pulse Generator/1 -> Sum1/1
  Constant/1 -> Sum1/2
  Sum2/1 -> Simulink-PS Converter/1
  Pulse Generator1/1 -> Sum2/1
  Constant1/1 -> Sum2/2
  connections:
  World Frame/RConn1 -- Solver Configuration/RConn1 -- Transform Sensor1/LConn1 -- Transform Sensor/LConn1 -- Mechanism Configuration/RConn1 -- Rigid Transform1/LConn1
  Rigid Transform2/RConn1 -- Prismatic Joint/LConn1
  Rigid Transform1/RConn1 -- Rigid Transform2/LConn1
  Link 1/LConn1 -- Revolute Joint/RConn1
  Hook - Payload/LConn1 -- Revolute Joint2/RConn1
  Payload/RConn1 -- External Force and Torque/RConn1 -- Transform Sensor1/RConn1 -- Hook - Payload/LConn2
  Link 2/LConn1 -- Revolute Joint3/RConn1
  Link 3/LConn1 -- Revolute Joint4/RConn1
  Revolute Joint3/LConn1 -- PM 1/RConn1 -- Link 1/LConn2
  Revolute Joint4/LConn1 -- PM 2/RConn1 -- Link 2/LConn2
  PM 3/RConn1 -- Revolute Joint5/LConn1 -- Link 3/LConn2
  Link 5/LConn2 -- PM 5/RConn1 -- Revolute Joint7/LConn1
  Revolute Joint6/LConn1 -- PM 4/RConn1 -- Link 4/LConn2
  Link 5/LConn1 -- Revolute Joint6/RConn1
  Link 4/LConn1 -- Revolute Joint5/RConn1
  Revolute Joint10/LConn1 -- PM 8/RConn1 -- Link 8/LConn2
  Link 7/LConn2 -- PM 7/RConn1 -- Revolute Joint9/LConn1
  Revolute Joint8/LConn1 -- PM 6/RConn1 -- Link 6/LConn2
  Link 9/LConn2 -- PM 9/RConn1 -- Revolute Joint11/LConn1
  Link 9/LConn1 -- Revolute Joint10/RConn1
  Link 8/LConn1 -- Revolute Joint9/RConn1
  Link 7/LConn1 -- Revolute Joint8/RConn1
  Link 6/LConn1 -- Revolute Joint7/RConn1
  Link 11/LConn2 -- PM 11/RConn1 -- Revolute Joint15/LConn1
  Revolute Joint14/LConn1 -- PM 10/RConn1 -- Link 10/LConn2
  Revolute Joint12/LConn1 -- PM 16/RConn1 -- Link 16/LConn2
  Revolute Joint16/LConn1 -- PM 12/RConn1 -- Link 12/LConn2
  Link 17/LConn2 -- PM 17/RConn1 -- Revolute Joint13/LConn1
  Link 15/LConn2 -- PM 15/RConn1 -- Revolute Joint19/LConn1
  Link 13/LConn2 -- PM 13/RConn1 -- Revolute Joint17/LConn1
  Revolute Joint18/LConn1 -- PM 14/RConn1 -- Link 14/LConn2
  Link 16/LConn1 -- Revolute Joint19/RConn1
  Link 11/LConn1 -- Revolute Joint14/RConn1
  Link 17/LConn1 -- Revolute Joint12/RConn1
  Link 12/LConn1 -- Revolute Joint15/RConn1
  Link 14/LConn1 -- Revolute Joint17/RConn1
  Link 15/LConn1 -- Revolute Joint18/RConn1
  Link 13/LConn1 -- Revolute Joint16/RConn1
  Link 18/LConn2 -- PM 18/RConn1 -- Revolute Joint22/LConn1
  Link 19/LConn2 -- Hook/RConn1 -- Revolute Joint2/LConn1
  Link 18/LConn1 -- Revolute Joint13/RConn1
  Link 10/LConn1 -- Revolute Joint11/RConn1
  Rigid Transform4/LConn1 -- Rigid Transform3/RConn1
  PS-Simulink Converter3/LConn1 -- Transform Sensor/RConn2
  PS-Simulink Converter4/LConn1 -- Transform Sensor/RConn3
  Transform Sensor1/RConn2 -- PS-Simulink Converter1/LConn1
  Transform Sensor1/RConn3 -- PS-Simulink Converter5/LConn1
  PS-Simulink Converter6/LConn1 -- Revolute Joint3/RConn2
  PS-Simulink Converter42/LConn1 -- Revolute Joint4/RConn2
  PS-Simulink Converter40/LConn1 -- Revolute Joint5/RConn2
  PS-Simulink Converter38/LConn1 -- Revolute Joint6/RConn2
  PS-Simulink Converter36/LConn1 -- Revolute Joint7/RConn2
  PS-Simulink Converter34/LConn1 -- Revolute Joint8/RConn2
  PS-Simulink Converter32/LConn1 -- Revolute Joint9/RConn2
  PS-Simulink Converter30/LConn1 -- Revolute Joint10/RConn2
  PS-Simulink Converter28/LConn1 -- Revolute Joint11/RConn2
  PS-Simulink Converter26/LConn1 -- Revolute Joint14/RConn2
  PS-Simulink Converter24/LConn1 -- Revolute Joint15/RConn2
  PS-Simulink Converter22/LConn1 -- Revolute Joint16/RConn2
  PS-Simulink Converter20/LConn1 -- Revolute Joint17/RConn2
  PS-Simulink Converter18/LConn1 -- Revolute Joint18/RConn2
  PS-Simulink Converter16/LConn1 -- Revolute Joint19/RConn2
  PS-Simulink Converter14/LConn1 -- Revolute Joint12/RConn2
  PS-Simulink Converter12/LConn1 -- Revolute Joint13/RConn2
  PS-Simulink Converter10/LConn1 -- Revolute Joint22/RConn2
  PS-Simulink Converter8/LConn1 -- Revolute Joint2/RConn2
  PS-Simulink Converter2/LConn1 -- Revolute Joint/RConn2
  Revolute Joint/RConn3 -- PS-Simulink Converter11/LConn1
  PS-Simulink Converter13/LConn1 -- Revolute Joint3/RConn3
  PS-Simulink Converter15/LConn1 -- Revolute Joint4/RConn3
  PS-Simulink Converter17/LConn1 -- Revolute Joint5/RConn3
  PS-Simulink Converter19/LConn1 -- Revolute Joint6/RConn3
  PS-Simulink Converter21/LConn1 -- Revolute Joint7/RConn3
  PS-Simulink Converter23/LConn1 -- Revolute Joint8/RConn3
  PS-Simulink Converter25/LConn1 -- Revolute Joint9/RConn3
  PS-Simulink Converter27/LConn1 -- Revolute Joint10/RConn3
  PS-Simulink Converter29/LConn1 -- Revolute Joint11/RConn3
  PS-Simulink Converter35/LConn1 -- Revolute Joint17/RConn3
  PS-Simulink Converter37/LConn1 -- Revolute Joint18/RConn3
  PS-Simulink Converter39/LConn1 -- Revolute Joint19/RConn3
  PS-Simulink Converter41/LConn1 -- Revolute Joint14/RConn3
  PS-Simulink Converter31/LConn1 -- Revolute Joint15/RConn3
  PS-Simulink Converter33/LConn1 -- Revolute Joint16/RConn3
  PS-Simulink Converter43/LConn1 -- Revolute Joint12/RConn3
  PS-Simulink Converter44/LConn1 -- Revolute Joint13/RConn3
  PS-Simulink Converter45/LConn1 -- Revolute Joint22/RConn3
  PS-Simulink Converter46/LConn1 -- Revolute Joint2/RConn3
  Link 19/LConn1 -- Revolute Joint22/RConn1
  Rigid Transform5/RConn1 -- Revolute Joint/LConn1
  Prismatic Joint/RConn1 -- Rigid Transform3/LConn1 -- Transform Sensor/RConn1 -- Cart/RConn1
  Rigid Transform4/RConn1 -- Rigid Transform5/LConn1
  External Force and Torque/LConn1 -- Simulink-PS Converter/RConn1
  Prismatic Joint/LConn2 -- Simulink-PS Converter1/RConn1

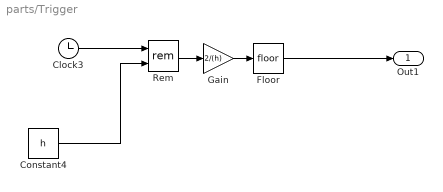
== system parts/Trigger ==
  Clock3 : Clock
  Constant4 : Constant  Value=h
  Floor : Rounding
  Gain : Gain  Gain=2/(h)
  Rem : Math  Operator=rem  SignedPower=on  SaturateOnIntegerOverflow=on
  Out1 : Outport
  wires:
  Rem/1 -> Gain/1
  Gain/1 -> Floor/1
  Constant4/1 -> Rem/2
  Clock3/1 -> Rem/1
  Floor/1 -> Out1/1

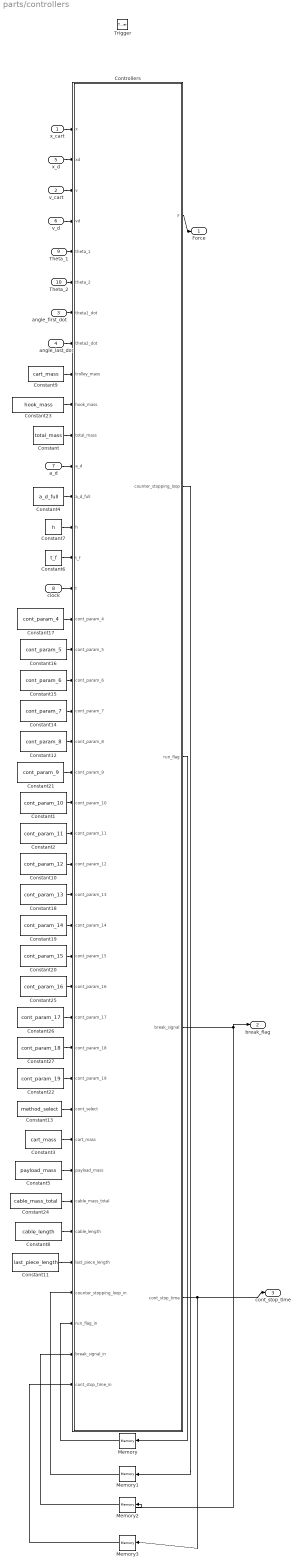
== system parts/controllers ==
  x_cart : Inport
  v_cart : Inport  Port=2
  angle_first_dot : Inport  Port=3
  angle_last_dot : Inport  Port=4
  x_d : Inport  Port=5
  v_d : Inport  Port=6
  a_d : Inport  Port=7
  clock : Inport  Port=8
  Theta_1 : Inport  Port=9
  Theta_2 : Inport  Port=10
  Trigger : TriggerPort  VariantControl=(inherit)
  Constant : Constant  Value=total_mass
  Constant1 : Constant  Value=cont_param_10
  Constant10 : Constant  Value=cont_param_12
  Constant11 : Constant  Value=last_piece_length
  Constant12 : Constant  Value=cont_param_8
  Constant13 : Constant  Value=method_select
  Constant14 : Constant  Value=cont_param_7
  Constant15 : Constant  Value=cont_param_6
  Constant16 : Constant  Value=cont_param_5
  Constant17 : Constant  Value=cont_param_4
  Constant18 : Constant  Value=cont_param_13
  Constant19 : Constant  Value=cont_param_14
  Constant2 : Constant  Value=cont_param_11
  Constant20 : Constant  Value=cont_param_15
  Constant21 : Constant  Value=cont_param_9
  Constant22 : Constant  Value=cont_param_19
  Constant23 : Constant  Value=hook_mass
  Constant24 : Constant  Value=cable_mass_total
  Constant25 : Constant  Value=cont_param_16
  Constant26 : Constant  Value=cont_param_17
  Constant27 : Constant  Value=cont_param_18
  Constant3 : Constant  Value=cart_mass
  Constant4 : Constant  Value=a_d_full
  Constant5 : Constant  Value=payload_mass
  Constant6 : Constant  Value=t_f
  Constant7 : Constant  Value=h
  Constant8 : Constant  Value=cable_length
  Constant9 : Constant  Value=cart_mass
  Controllers : MATLAB Function  TreatAsAtomicUnit=on
  Memory : Memory  InitialCondition=1  InheritSampleTime=on
  Memory1 : Memory  InheritSampleTime=on
  Memory2 : Memory  InheritSampleTime=on
  Memory3 : Memory  InitialCondition=t_f  InheritSampleTime=on
  Force : Outport
  break_flag : Outport  Port=2
  cont_stop_time : Outport  Port=3
  wires:
  Constant/1 -> Controllers/11(total_mass)
  Constant13/1 -> Controllers/33(cont_select)
  Constant21/1 -> Controllers/22(cont_param_9)
  Constant12/1 -> Controllers/21(cont_param_8)
  Constant15/1 -> Controllers/19(cont_param_6)
  Constant16/1 -> Controllers/18(cont_param_5)
  Constant17/1 -> Controllers/17(cont_param_4)
  Controllers/1(F) -> Force/1
  v_d/1 -> Controllers/4(vd)
  a_d/1 -> Controllers/12(a_d)
  clock/1 -> Controllers/16(t)
  Theta_1/1 -> Controllers/5(theta_1)
  Theta_2/1 -> Controllers/6(theta_2)
  x_d/1 -> Controllers/2(xd)
  v_cart/1 -> Controllers/3(v)
  x_cart/1 -> Controllers/1(x)
  Constant24/1 -> Controllers/36(cable_mass_total)
  Constant9/1 -> Controllers/9(trolley_mass)
  Constant4/1 -> Controllers/13(a_d_full)
  Constant7/1 -> Controllers/14(h)
  Constant6/1 -> Controllers/15(t_f)
  Constant23/1 -> Controllers/10(hook_mass)
  angle_first_dot/1 -> Controllers/7(theta1_dot)
  angle_last_dot/1 -> Controllers/8(theta2_dot)
  Constant14/1 -> Controllers/20(cont_param_7)
  Controllers/2(counter_stopping_loop) -> Memory1/1
  Memory/1 -> Controllers/40(run_flag_in)
  Memory1/1 -> Controllers/39(counter_stopping_loop_in)
  Controllers/4(break_signal) -> Memory2/1, break_flag/1
  Controllers/3(run_flag) -> Memory/1
  Memory2/1 -> Controllers/41(break_signal_in)
  Controllers/5(cont_stop_time) -> cont_stop_time/1, Memory3/1
  Memory3/1 -> Controllers/42(cont_stop_time_in)
  Constant1/1 -> Controllers/23(cont_param_10)
  Constant2/1 -> Controllers/24(cont_param_11)
  Constant3/1 -> Controllers/34(cart_mass)
  Constant5/1 -> Controllers/35(payload_mass)
  Constant8/1 -> Controllers/37(cable_length)
  Constant11/1 -> Controllers/38(last_piece_length)
  Constant10/1 -> Controllers/25(cont_param_12)
  Constant18/1 -> Controllers/26(cont_param_13)
  Constant19/1 -> Controllers/27(cont_param_14)
  Constant20/1 -> Controllers/28(cont_param_15)
  Constant25/1 -> Controllers/29(cont_param_16)
  Constant26/1 -> Controllers/30(cont_param_17)
  Constant27/1 -> Controllers/31(cont_param_18)
  Constant22/1 -> Controllers/32(cont_param_19)
